simulink model "AppDesign3"  (R2019a)
settings: Solver=VariableStepAuto  StartTime=0.0  StopTime=10.0  RelTol=1e-3
settings Model: Creator=G5  LastModifiedBy=G5

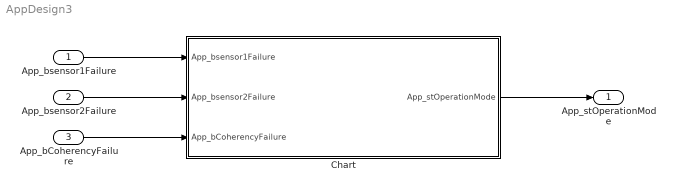
== system AppDesign3 ==
  App_bsensor1Failure : Inport
  App_bsensor2Failure : Inport  Port=2
  App_bCoherencyFailure : Inport  Port=3
  Chart : Stateflow chart  BlockKeywords=__PRM__SERIALIZED__DATA__:Stateflow Chart,Stateflow Diagram  TreatAsAtomicUnit=on
  App_stOperationMode : Outport  OutDataTypeStr=Enum: App_Modes
  wires:
  App_bsensor1Failure/1 -> Chart/1(App_bsensor1Failure)
  App_bsensor2Failure/1 -> Chart/2(App_bsensor2Failure)
  App_bCoherencyFailure/1 -> Chart/3(App_bCoherencyFailure)
  Chart/1(App_stOperationMode) -> App_stOperationMode/1

== stateflow chart AppDesign3/Chart ==
  (default) -> (junction 64) : % Modes
  (junction 64) -> (junction 65) [order 1] : [App_bCoherencyFailure]
  (junction 64) -> (junction 66) [order 2]
  (junction 65) -> (junction 73) : {App_stOperationMode = App_Modes.Failure;}
  (junction 66) -> (junction 67) [order 1] : [App_bsensor2Failure && ~App_bsensor1Failure]
  (junction 66) -> (junction 68) [order 2]
  (junction 67) -> (junction 72) : {App_stOperationMode = App_Modes.Downgraded_Sen_1;}
  (junction 68) -> (junction 69) [order 1] : [App_bsensor1Failure && ~App_bsensor2Failure]
  (junction 68) -> (junction 70) [order 2] : {App_stOperationMode = App_Modes.Normal;}
  (junction 69) -> (junction 71) : {App_stOperationMode = App_Modes.Downgraded_Sen_2;}
  (junction 71) -> (junction 70)
  (junction 72) -> (junction 71)
  (junction 73) -> (junction 72)
  (junction 70) -> (junction 74)
  data: App_bsensor1Failure input; App_bsensor2Failure input; App_bCoherencyFailure input; App_stOperationMode output
